simulink model "subsystem"  (R2020b)
settings: Solver=VariableStepAuto  StartTime=0.0  StopTime=10.0  RelTol=1e-3
settings Model: Creator=ADMIN  LastModifiedBy=ADMIN

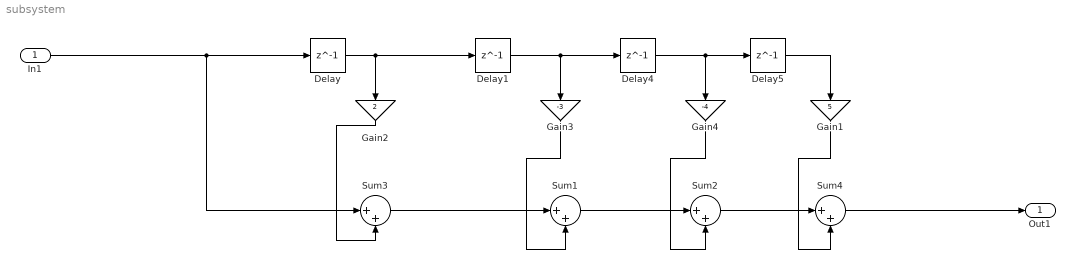
== system subsystem ==
  In1 : Inport  OutDataTypeStr=double  PortDimensions=1  SampleTime=[0,1]
  Delay{,1,4..5} (4 alike) : Delay  DelayLength=1
  Gain1 : Gain  Gain=5
  Gain2 : Gain  Gain=2
  Gain3 : Gain  Gain=-3
  Gain4 : Gain  Gain=-4
  Sum{1..4} (4 alike) : Sum  Inputs=|++
  Out1 : Outport  OutDataTypeStr=double  PortDimensions=1  SampleTime=[0,1]
  wires:
  Delay4/1 -> Delay5/1, Gain4/1
  In1/1 -> Delay/1, Sum3/1
  Sum4/1 -> Out1/1
  Delay5/1 -> Gain1/1
  Delay/1 -> Delay1/1, Gain2/1
  Gain2/1 -> Sum3/2
  Gain1/1 -> Sum4/2
  Sum1/1 -> Sum2/1
  Gain3/1 -> Sum1/2
  Sum3/1 -> Sum1/1
  Sum2/1 -> Sum4/1
  Gain4/1 -> Sum2/2
  Delay1/1 -> Delay4/1, Gain3/1
